simulink model "TRMS_sim_SFV2"  (R2021a)
settings: Solver=VariableStepAuto  StartTime=0.0  StopTime=600  MaxStep=1e-2  RelTol=1e-3
values from neighbouring files (symbols this model uses):
  K =     [controllerV22OrigLMI.mat]
  Ts = 0.01    [BuildGridCustom.m]    (also in workspacesetup.m = 0.02)
  Weh = c2d(We,Ts,'Tustin')    [BuildGridCustom.m]
  Wev = c2d(We,Ts,'Tustin')    [BuildGridCustom.m]
  Wewh = c2d(We,Ts,'Tustin')    [BuildGridCustom.m]
  Wewv = c2d(We,Ts,'Tustin')    [BuildGridCustom.m]
  Wuh = c2d(Wu,Ts,'Tustin')    [BuildGridCustom.m]
  Wuv = c2d(Wu,Ts,'Tustin')    [BuildGridCustom.m]
undefined symbols (not defined in the file or in its folder): GridK_PL_SFV2, TRMS
settings Model: Creator=ariel  LastModifiedBy=ariel

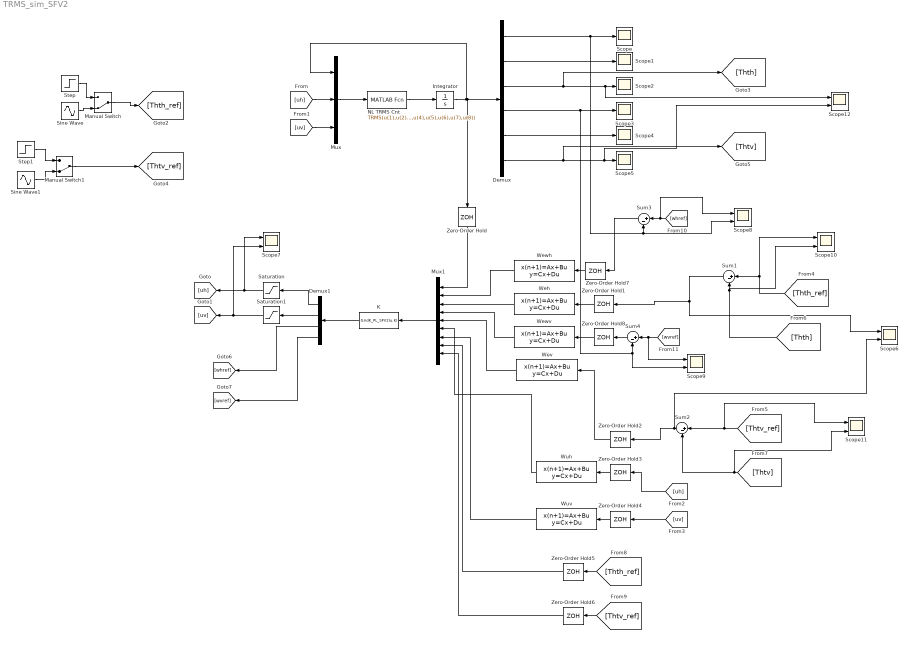
== system TRMS_sim_SFV2 ==
  Demux : Demux  Outputs=6
  Demux1 : Demux
  Integrator : Integrator
  K : MATLABFcn  MATLABFcn=GridK_PL_SFV2(u,K)  OutputDimensions=4
  Manual Switch : ManualSwitch  CurrentSetting=0
  Manual Switch1 : ManualSwitch  CurrentSetting=0
  Mux : Mux  Inputs=3
  Mux1 : Mux  Inputs=9
      settings: DisplayOption=signals
  NL TRMS Cnt : MATLABFcn  MATLABFcn=TRMS(u(1),u(2),u(3),u(4),u(5),u(6),u(7),u(8))  OutputDimensions=6
  Saturation : Saturate  UpperLimit=2.5  LowerLimit=-2.5
  Saturation1 : Saturate  UpperLimit=2  LowerLimit=-2
  Scope{,1..5} (6 alike) : Scope
  Scope{6..12} (7 alike) : Scope  NumInputPorts=2
  Sine Wave : Sin  Amplitude=0.7  Frequency=2*pi*(1/115)  Phase=0.16  SampleTime=0
  Sine Wave1 : Sin  Amplitude=0.5  Bias=-0.2  Frequency=2*pi*(1/90)  Phase=-0.3  SampleTime=0
  Step : Step  Time=170  Before=-0.7  After=0.5  SampleTime=10
  Step1 : Step  Time=90  Before=-0.7  After=0.1  SampleTime=10
  Sum{1..4} (4 alike) : Sum  Inputs=|+-
  Weh : DiscreteStateSpace  A=Weh.A  B=Weh.B  D=0  SampleTime=Ts
  Wev : DiscreteStateSpace  A=Wev.A  B=Wev.B  D=0  SampleTime=Ts
  Wewh : DiscreteStateSpace  A=Wewh.A  B=Wewh.B  D=0  SampleTime=Ts
  Wewv : DiscreteStateSpace  A=Wewv.A  B=Wewv.B  D=0  SampleTime=Ts
  Wuh : DiscreteStateSpace  A=Wuh.A  B=Wuh.B  D=0  SampleTime=Ts
  Wuv : DiscreteStateSpace  A=Wuv.A  B=Wuv.B  D=0  SampleTime=Ts
  Zero-Order Hold{,1..8} (9 alike) : ZeroOrderHold  SampleTime=Ts
  wires:
  NL TRMS Cnt/1 -> Integrator/1
  Mux/1 -> NL TRMS Cnt/1
  Integrator/1 -> Zero-Order Hold/1, Demux/1, Mux/1
  Demux/1 -> Scope8/2, Sum3/2, Scope/1
  Demux/5 -> Scope4/1
  Demux/4 -> Scope9/2, Sum4/2, Scope3/1
  Demux/3 -> [Thth], Scope12/1, Scope2/1
  Demux/2 -> Scope1/1
  Mux1/1 -> K/1
  K/1 -> Demux1/1
  Demux1/1 -> Saturation/1
  Demux1/2 -> Saturation1/1
  [uh] -> Mux/2
  [uv] -> Mux/3
  [uh] -> Zero-Order Hold3/1
  [uv] -> Zero-Order Hold4/1
  Demux/6 -> Scope12/2, Scope5/1, [Thtv]
  [Thth_ref] -> Scope10/1, Sum1/1
  [Thth] -> Scope10/2, Sum1/2
  Sum1/1 -> Scope6/1, Zero-Order Hold1/1
  [Thtv_ref] -> Scope11/1, Sum2/1
  Sum2/1 -> Zero-Order Hold2/1, Scope6/2
  [Thtv] -> Scope11/2, Sum2/2
  Saturation/1 -> Scope7/1, [uh]
  Saturation1/1 -> Scope7/2, [uv]
  Zero-Order Hold/1 -> Mux1/1
  Zero-Order Hold1/1 -> Weh/1
  Zero-Order Hold2/1 -> Wev/1
  Zero-Order Hold3/1 -> Wuh/1
  Zero-Order Hold4/1 -> Wuv/1
  [Thth_ref] -> Zero-Order Hold5/1
  [Thtv_ref] -> Zero-Order Hold6/1
  Wewh/1 -> Mux1/2
  Weh/1 -> Mux1/3
  Wewv/1 -> Mux1/4
  Wev/1 -> Mux1/5
  Wuh/1 -> Mux1/6
  Wuv/1 -> Mux1/7
  Zero-Order Hold5/1 -> Mux1/8
  Zero-Order Hold6/1 -> Mux1/9
  Demux1/3 -> [whref]
  Demux1/4 -> [wvref]
  [whref] -> Scope8/1, Sum3/1
  Sum3/1 -> Zero-Order Hold7/1
  Zero-Order Hold7/1 -> Wewh/1
  Zero-Order Hold8/1 -> Wewv/1
  Sum4/1 -> Zero-Order Hold8/1
  [wvref] -> Scope9/1, Sum4/1
  Manual Switch/1 -> [Thth_ref]
  Sine Wave/1 -> Manual Switch/2
  Step/1 -> Manual Switch/1
  Sine Wave1/1 -> Manual Switch1/2
  Step1/1 -> Manual Switch1/1
  Manual Switch1/1 -> [Thtv_ref]
